simulink model "Project1Part2_"  (R2023b)
settings: Solver=ode1  StartTime=0.0  StopTime=25  FixedStep=0.1  RelTol=1e-3
values from neighbouring files (symbols this model uses):
  A = 1    [Project1Week2.m]    (also in ProjectWeek1.m; Project_1.m = 4)
  F = 0    [Project1Final.m]
  isSin = 1    [Project1Final.m]
  w_0 = 1    [Project1Week2.m]    (also in ProjectWeek1.m; Project_1.m)
undefined symbols (not defined in the file or in its folder): b1, b2, J1, J2, k
settings Model: Creator=Julian Tan  LastModifiedBy=julia

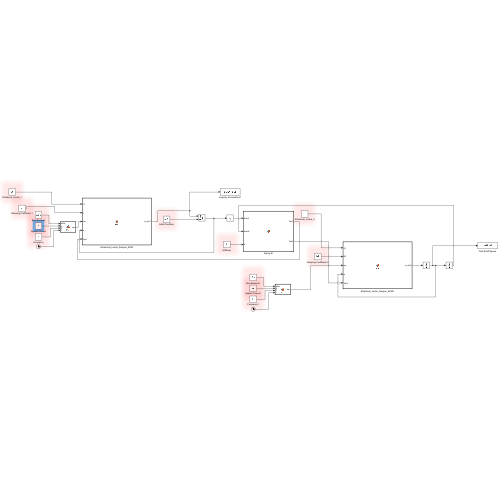
[thumbnail: Simulink's stored preview of the top-level diagram]
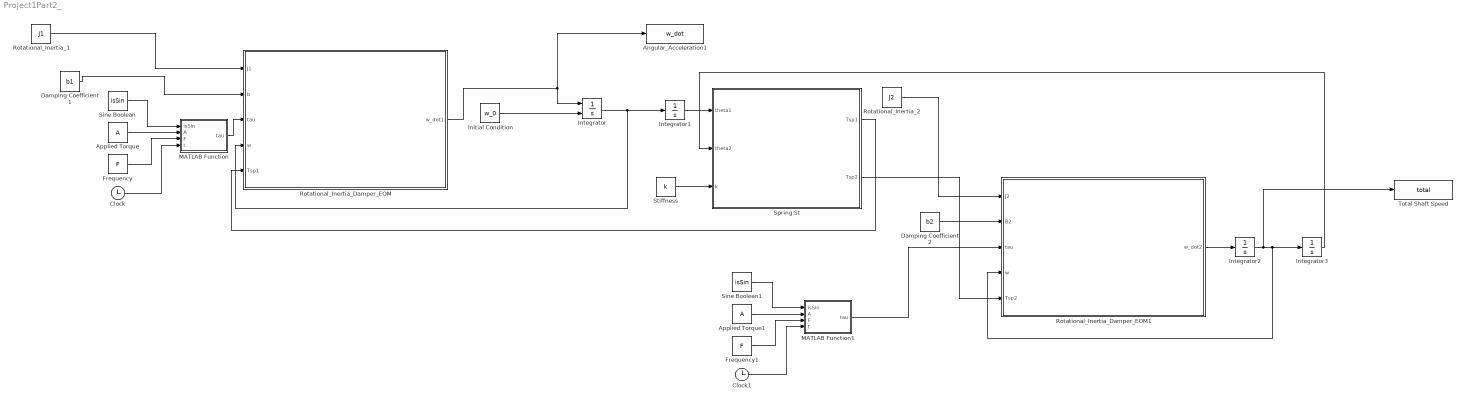
== system Project1Part2_ ==
  Angular_Acceleration1 : ToWorkspace  VariableName=w_dot  SaveFormat=Timeseries  SampleTime=-1
  Applied Torque : Constant  Value=A
  Applied Torque1 : Constant  Value=A
  Clock : Clock
  Clock1 : Clock
  Damping Coefficient 1 : Constant  Value=b1
  Damping Coefficient 2 : Constant  Value=b2
  Frequency : Constant  Value=F
  Frequency1 : Constant  Value=F
  Initial Condition : Constant  Value=w_0
  Integrator : Integrator  InitialConditionSource=external  LimitOutput=on  UpperSaturationLimit=10
  Integrator1 : Integrator
  Integrator2 : Integrator
  Integrator3 : Integrator
  MATLAB Function : MATLAB Function  TreatAsAtomicUnit=on
  MATLAB Function1 : MATLAB Function  TreatAsAtomicUnit=on
  Rotational_Inertia_1 : Constant  Value=J1
  Rotational_Inertia_2 : Constant  Value=J2
  Rotational_Inertia_Damper_EOM : MATLAB Function  TreatAsAtomicUnit=on
  Rotational_Inertia_Damper_EOM1 : MATLAB Function  TreatAsAtomicUnit=on
  Sine Boolean : Constant  Value=isSin
  Sine Boolean1 : Constant  Value=isSin
  Spring St : MATLAB Function  TreatAsAtomicUnit=on
  Stiffness : Constant  Value=k
  "Total Shaft Speed " : ToWorkspace  VariableName=total  SaveFormat=Timeseries  SampleTime=-1
  wires:
  Rotational_Inertia_Damper_EOM/1(w_dot1) -> Angular_Acceleration1/1, Integrator/1
  Applied Torque/1 -> MATLAB Function/2(A)
  Initial Condition/1 -> Integrator/2
  Damping Coefficient 1/1 -> Rotational_Inertia_Damper_EOM/2(b)
  Integrator/1 -> Integrator1/1, Rotational_Inertia_Damper_EOM/4(w)
  Rotational_Inertia_1/1 -> Rotational_Inertia_Damper_EOM/1(J1)
  Clock/1 -> MATLAB Function/4(t)
  Frequency/1 -> MATLAB Function/3(F)
  MATLAB Function/1(tau) -> Rotational_Inertia_Damper_EOM/3(tau)
  Sine Boolean/1 -> MATLAB Function/1(isSin)
  Stiffness/1 -> Spring St/3(k)
  Integrator1/1 -> Spring St/1(theta1)
  Rotational_Inertia_Damper_EOM1/1(w_dot2) -> Integrator2/1
  Integrator2/1 -> "Total Shaft Speed "/1, Rotational_Inertia_Damper_EOM1/4(w), Integrator3/1
  Integrator3/1 -> Spring St/2(theta2)
  Spring St/2(Tsp2) -> Rotational_Inertia_Damper_EOM1/5(Tsp2)
  Spring St/1(Tsp1) -> Rotational_Inertia_Damper_EOM/5(Tsp1)
  Rotational_Inertia_2/1 -> Rotational_Inertia_Damper_EOM1/1(J2)
  Damping Coefficient 2/1 -> Rotational_Inertia_Damper_EOM1/2(B2)
  Sine Boolean1/1 -> MATLAB Function1/1(isSin)
  Frequency1/1 -> MATLAB Function1/3(F)
  Clock1/1 -> MATLAB Function1/4(t)
  Applied Torque1/1 -> MATLAB Function1/2(A)
  MATLAB Function1/1(tau) -> Rotational_Inertia_Damper_EOM1/3(tau)

== matlab function Project1Part2_/MATLAB Function ==
  data: isSin input; tau output; A input; F input; t input
function tau = fcn(isSin, A, F, t)

if isSin == 0
    tau = A;
else
    tau = A*sin(F*t);
end

== matlab function Project1Part2_/Rotational_Inertia_Damper_EOM ==
  data: J1 input; w_dot1 output; b input; tau input; w input; Tsp1 input
function w_dot1 = fcn(J1, b, tau, w, Tsp1)

tau_damped = b*w;
w_dot1 = (1/J1)*(tau - tau_damped);

end

== matlab function Project1Part2_/Spring St ==
  data: theta1 input; Tsp1 output; theta2 input; Tsp2 output; k input
function [Tsp1,Tsp2] = f(theta1,theta2, k)

Tsp1 = -(K * (theta1 - theta2);


Tsp2 = K * (theta1 - theta2;

end

== matlab function Project1Part2_/Rotational_Inertia_Damper_EOM1 ==
  data: J2 input; w_dot2 output; B2 input; tau input; w input; Tsp2 input
function w_dot2 = fcn(J2, B2, tau, w, Tsp2)

tau_damped = b*w;
w_dot2 = (1/J2)*(Tsp2-tau_damped);

end

== matlab function Project1Part2_/MATLAB Function1 ==
  data: isSin input; tau output; A input; F input; t input
function tau = fcn(isSin, A, F, t)

if isSin == 0
    tau = A;
else
    tau = A*sin(F*t);
end
